simulink model "SimPIDlat"  (R2022a)
settings: Solver=VariableStepAuto  StartTime=0.0  StopTime=15  RelTol=1e-3
undefined symbols (not defined in the file): g_p, Kd, Ki, Kp
libraries: slpidlib x2, simulink x1
settings Model: Creator=danie  LastModifiedBy=Wulics
settings SolverCC: AlgebraicLoopSolver=TrustRegion
settings RTWCC: DLArmComputeVersion=19.05

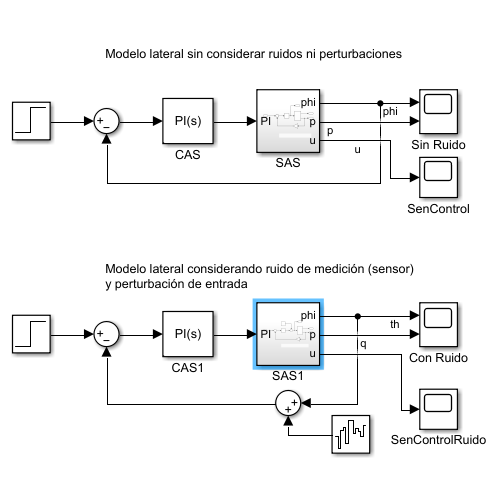
[thumbnail: Simulink's stored preview of the top-level diagram]
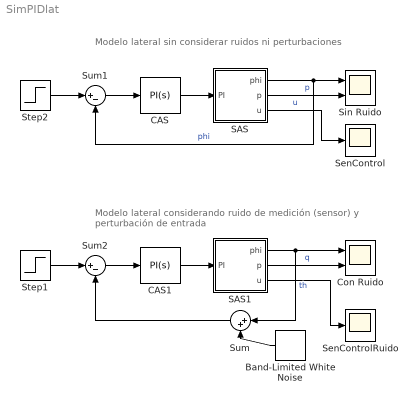
== system SimPIDlat ==
  note: Modelo lateral sin considerar ruidos ni perturbaciones
  note: Modelo lateral considerando ruido de medición (sensor)
      | y perturbación de entrada
  Band-Limited White Noise : simulink/Sources/Band-Limited White Noise  Cov=[0.001]  Ts=0.1  seed=[23341]
  CAS : slpidlib/PID Controller  Controller=PI  Form=Parallel  TimeDomain=Continuous-time  UseExternalTs=off  SampleTime=-1  IntegratorMethod=Forward Euler  FilterMethod=Forward Euler  ControllerParametersSource=internal  P=Kp  I=Ki  UseKiTs=off  D=0  N=100  UseFilter=on  TunerSelectOption=Transfer Function Based (PID Tuner App)  InitialConditionSource=internal  InitialConditionForIntegrator=0  InitialConditionForFilter=0  DifferentiatorICPrevScaledInput=0  ExternalReset=none  TrackingMode=off  Kt=1  LimitOutput=off  SatLimitsSource=internal  UpperSaturationLimit=inf  LowerSaturationLimit=-inf  LinearizeAsGain=on  AntiWindupMode=none  Kb=1  POutMin=[]  POutMax=[]  IOutMin=[]  IOutMax=[]  DOutMin=[]  DOutMax=[]  NOutMin=[]  NOutMax=[]  SumOutMin=[]  SumOutMax=[]  SaturationOutMin=[]  SaturationOutMax=[]  PParamMin=[]  PParamMax=[]  IParamMin=[]  IParamMax=[]  DParamMin=[]  DParamMax=[]  NParamMin=[]  NParamMax=[]  KbParamMin=[]  KbParamMax=[]  KtParamMin=[]  KtParamMax=[]  KbOutMin=[]  KbOutMax=[]  KtOutMin=[]  KtOutMax=[]  IntegratorOutMin=[]  IntegratorOutMax=[]  FilterOutMin=[]  FilterOutMax=[]  SumI1OutMin=[]  SumI1OutMax=[]  SumI2OutMin=[]  SumI2OutMax=[]  SumI3OutMin=[]  SumI3OutMax=[]  SumI4OutMin=[]  SumI4OutMax=[]  SumDOutMin=[]  SumDOutMax=[]  DifferentiatorOutMin=[]  DifferentiatorOutMax=[]  FilterDiffOutCoefMin=[]  FilterDiffOutCoefMax=[]  ReciprocalOutMin=[]  ReciprocalOutMax=[]  SumDenOutMin=[]  SumDenOutMax=[]  SumNumOutMin=[]  SumNumOutMax=[]  DivideOutMin=[]  DivideOutMax=[]  UdiffTsProdOutMin=[]  UdiffTsProdOutMax=[]  NTsProdOutMin=[]  NTsProdOutMax=[]  UintegralTsProdOutMin=[]  UintegralTsProdOutMax=[]  UngainTsProdOutMin=[]  UngainTsProdOutMax=[]  IntegratorContinuousStateAttributes=''  IntegratorStateMustResolveToSignalObject=off  IntegratorRTWStateStorageClass=Auto  FilterContinuousStateAttributes=''  FilterStateMustResolveToSignalObject=off  FilterRTWStateStorageClass=Auto  ParallelPVariant=InternalParameters  IdealPVariant=Disabled  IVariant=InternalParameters  DVariant=Disabled  IntegratorVariant=Continuous  SatVariant=Disabled  AWVariant=Passthrough  PCopyVariant=Disabled  TRVariant=Disabled  FdbkBlocksVariant=Forward  IdealPFdbkVariant=Disabled  SatFdbkVariant=Disabled  DerivativeFilterVariant=Disabled  NVariant=Disabled  NCopyVariant=Disabled_SignalSpec  FilterICVariant=Disabled  IntegratorICVariant=InternalICs  ExternalResetVariant=Disabled  TRSumVariant=Passthrough  SumFdbkVariant=Disabled  SumVariant=Sum_PI  TsampFilterVariant=InternalTs  TsampNgainVariant=Passthrough  TsampIntegralVariant=Passthrough  ExternalSaturationOutDataTypeStr=Inherit: Same as second input  aMode=0
  CAS1 : slpidlib/PID Controller  Controller=PI  Form=Parallel  TimeDomain=Continuous-time  UseExternalTs=off  SampleTime=-1  IntegratorMethod=Forward Euler  FilterMethod=Forward Euler  ControllerParametersSource=internal  P=Kp  I=Ki  UseKiTs=off  D=0  N=100  UseFilter=on  TunerSelectOption=Transfer Function Based (PID Tuner App)  InitialConditionSource=internal  InitialConditionForIntegrator=0  InitialConditionForFilter=0  DifferentiatorICPrevScaledInput=0  ExternalReset=none  TrackingMode=off  Kt=1  LimitOutput=off  SatLimitsSource=internal  UpperSaturationLimit=inf  LowerSaturationLimit=-inf  LinearizeAsGain=on  AntiWindupMode=none  Kb=1  POutMin=[]  POutMax=[]  IOutMin=[]  IOutMax=[]  DOutMin=[]  DOutMax=[]  NOutMin=[]  NOutMax=[]  SumOutMin=[]  SumOutMax=[]  SaturationOutMin=[]  SaturationOutMax=[]  PParamMin=[]  PParamMax=[]  IParamMin=[]  IParamMax=[]  DParamMin=[]  DParamMax=[]  NParamMin=[]  NParamMax=[]  KbParamMin=[]  KbParamMax=[]  KtParamMin=[]  KtParamMax=[]  KbOutMin=[]  KbOutMax=[]  KtOutMin=[]  KtOutMax=[]  IntegratorOutMin=[]  IntegratorOutMax=[]  FilterOutMin=[]  FilterOutMax=[]  SumI1OutMin=[]  SumI1OutMax=[]  SumI2OutMin=[]  SumI2OutMax=[]  SumI3OutMin=[]  SumI3OutMax=[]  SumI4OutMin=[]  SumI4OutMax=[]  SumDOutMin=[]  SumDOutMax=[]  DifferentiatorOutMin=[]  DifferentiatorOutMax=[]  FilterDiffOutCoefMin=[]  FilterDiffOutCoefMax=[]  ReciprocalOutMin=[]  ReciprocalOutMax=[]  SumDenOutMin=[]  SumDenOutMax=[]  SumNumOutMin=[]  SumNumOutMax=[]  DivideOutMin=[]  DivideOutMax=[]  UdiffTsProdOutMin=[]  UdiffTsProdOutMax=[]  NTsProdOutMin=[]  NTsProdOutMax=[]  UintegralTsProdOutMin=[]  UintegralTsProdOutMax=[]  UngainTsProdOutMin=[]  UngainTsProdOutMax=[]  IntegratorContinuousStateAttributes=''  IntegratorStateMustResolveToSignalObject=off  IntegratorRTWStateStorageClass=Auto  FilterContinuousStateAttributes=''  FilterStateMustResolveToSignalObject=off  FilterRTWStateStorageClass=Auto  ParallelPVariant=InternalParameters  IdealPVariant=Disabled  IVariant=InternalParameters  DVariant=Disabled  IntegratorVariant=Continuous  SatVariant=Disabled  AWVariant=Passthrough  PCopyVariant=Disabled  TRVariant=Disabled  FdbkBlocksVariant=Forward  IdealPFdbkVariant=Disabled  SatFdbkVariant=Disabled  DerivativeFilterVariant=Disabled  NVariant=Disabled  NCopyVariant=Disabled_SignalSpec  FilterICVariant=Disabled  IntegratorICVariant=InternalICs  ExternalResetVariant=Disabled  TRSumVariant=Passthrough  SumFdbkVariant=Disabled  SumVariant=Sum_PI  TsampFilterVariant=InternalTs  TsampNgainVariant=Passthrough  TsampIntegralVariant=Passthrough  ExternalSaturationOutDataTypeStr=Inherit: Same as second input  aMode=0
  Con Ruido : Scope  NumInputPorts=2
  SAS : Subsystem
  SAS1 : Subsystem
  SenControl : Scope
  SenControlRuido : Scope
  Sin Ruido : Scope  NumInputPorts=2
  Step1 : Step  Time=0  After=40  SampleTime=0
  Step2 : Step  Time=0  After=40  SampleTime=0
  Sum : Sum  Inputs=|++
  Sum1 : Sum  Inputs=|+-
  Sum2 : Sum  Inputs=|+-
  wires:
  Sum1/1 -> CAS/1
  SAS/1(phi) -> Sin Ruido/1, Sum1/2  "phi"
  CAS/1 -> SAS/1(PI)
  Step2/1 -> Sum1/1
  Step1/1 -> Sum2/1
  CAS1/1 -> SAS1/1(PI)
  SAS1/2(p) -> Con Ruido/2  "q"
  SAS1/1(phi) -> Sum/1, Con Ruido/1  "th"
  Sum2/1 -> CAS1/1
  Band-Limited White Noise/1 -> Sum/2
  Sum/1 -> Sum2/2
  SAS/3(u) -> SenControl/1  "u"
  SAS1/3(u) -> SenControlRuido/1
  SAS/2(p) -> Sin Ruido/2  "p"

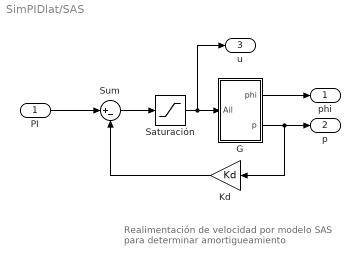
== system SimPIDlat/SAS ==
  note: Realimentación de velocidad por modelo SAS
      | para determinar amortigueamiento
  PI : Inport
  G : Subsystem
  Kd : Gain  Gain=Kd
  Saturación : Saturate  UpperLimit=30  LowerLimit=-30
  Sum : Sum  Inputs=|+-
  phi : Outport
  p : Outport  Port=2
  u : Outport  Port=3
  wires:
  G/2(p) -> p/1, Kd/1
  Kd/1 -> Sum/2
  G/1(phi) -> phi/1
  Sum/1 -> Saturación/1
  PI/1 -> Sum/1
  Saturación/1 -> u/1, G/1(Ail)

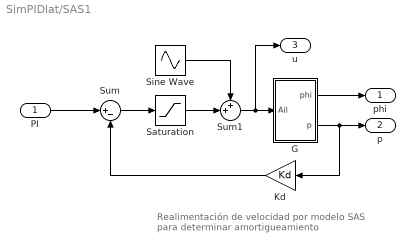
== system SimPIDlat/SAS1 ==
  note: Realimentación de velocidad por modelo SAS
      | para determinar amortigueamiento
  PI : Inport
  G : Subsystem
  Kd : Gain  Gain=Kd
  Saturation : Saturate  UpperLimit=30  LowerLimit=-30
  Sine Wave : Sin  Frequency=12*pi  SampleTime=0
  Sum : Sum  Inputs=|+-
  Sum1 : Sum  Inputs=++|
  phi : Outport
  p : Outport  Port=2
  u : Outport  Port=3
  wires:
  PI/1 -> Sum/1
  Sum/1 -> Saturation/1
  G/1(phi) -> phi/1
  Kd/1 -> Sum/2
  G/2(p) -> Kd/1, p/1
  Sine Wave/1 -> Sum1/1
  Sum1/1 -> u/1, G/1(Ail)
  Saturation/1 -> Sum1/2

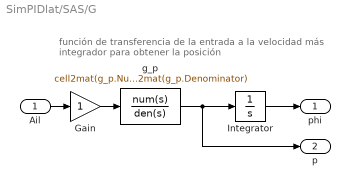
== system SimPIDlat/SAS/G ==
  note: función de transferencia de la entrada a la velocidad más
      | integrador para obtener la posición
  Ail : Inport
  Gain : Gain
  Integrator : Integrator
  g_p : TransferFcn  Numerator=cell2mat(g_p.Numerator)  Denominator=cell2mat(g_p.Denominator)
  phi : Outport
  p : Outport  Port=2
  wires:
  g_p/1 -> p/1, Integrator/1
  Integrator/1 -> phi/1
  Gain/1 -> g_p/1
  Ail/1 -> Gain/1

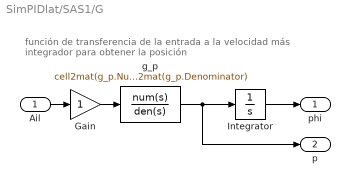
== system SimPIDlat/SAS1/G ==
  note: función de transferencia de la entrada a la velocidad más
      | integrador para obtener la posición
  Ail : Inport
  Gain : Gain
  Integrator : Integrator
  g_p : TransferFcn  Numerator=cell2mat(g_p.Numerator)  Denominator=cell2mat(g_p.Denominator)
  phi : Outport
  p : Outport  Port=2
  wires:
  Ail/1 -> Gain/1
  Gain/1 -> g_p/1
  Integrator/1 -> phi/1
  g_p/1 -> Integrator/1, p/1
